simulink model "sensorFusionOffline"  (Simulink 7.8)
settings: Solver=FixedStepDiscrete  StartTime=0.0  StopTime=endTime  FixedStep=0.005  MaxStep=0.005  RelTol=1e-3
undefined symbols (not defined in the file or in its folder): EGOSF_CompassHeadingCov, EGOSF_DetectionNorthMax, EGOSF_DetectionNorthMin, EGOSF_HeadingVelocityLimit, EGOSF_LatAccCov, EGOSF_LonAccCov, EGOSF_LonSpeedCov, EGOSF_OutlierDetection, EGOSF_PhiCov, EGOSF_PhiScale, EGOSF_Pproc, EGOSF_SteeringRatio, EGOSF_UTMZone, EGOSF_YawRateCov
libraries: powerlib_meascontrol x1
settings Model: Creator=hultr  LastModifiedBy=mdv91
settings DataIOCC: SignalLoggingSaveFormat=Dataset
settings OptimizationCC: ExpressionDepthLimit=128
settings DebuggingCC: UnderspecifiedInitializationDetection=Simplified  MergeDetectMultiDrivingBlocksExec=error  InheritedTsInSrcMsg=none  BusObjectLabelMismatch=none  StateNameClashWarn=none
settings CodeAppCC: CustomSymbolStrType=$N$R$M_T
settings GRTTargetCC: TargetFunctionLibrary=C89/C90 (ANSI)

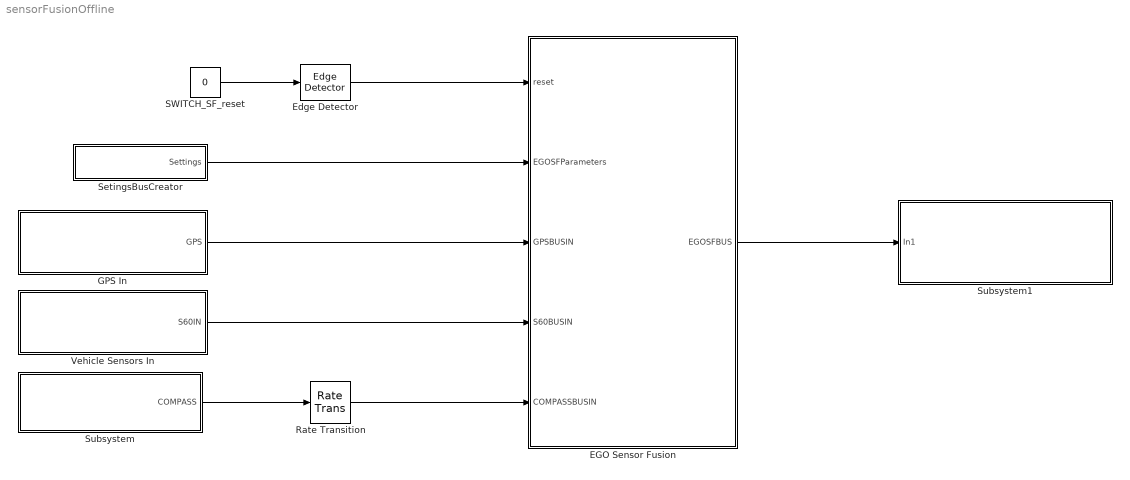
== system sensorFusionOffline ==
  EGO Sensor Fusion : MATLAB Function  TreatAsAtomicUnit=on  SystemSampleTime=0.025
      settings: PermitHierarchicalResolution=ParametersOnly
  Edge Detector : powerlib_meascontrol/Logic/Edge Detector  model=Rising  ic=0  Ts=-1
  GPS In : Subsystem
  Rate Transition : RateTransition
  SWITCH_SF_reset : Constant  Value=0  SampleTime=-1
  SetingsBusCreator : Subsystem
  Subsystem : Subsystem  TreatAsAtomicUnit=on  SystemSampleTime=0.1
  Subsystem1 : Subsystem
  Vehicle Sensors In : Subsystem
  wires:
  Subsystem/1("COMPASS ") -> Rate Transition/1
  GPS In/1(GPS) -> EGO Sensor Fusion/3(GPSBUSIN)
  Vehicle Sensors In/1(S60IN) -> EGO Sensor Fusion/4(S60BUSIN)
  SWITCH_SF_reset/1 -> Edge Detector/1
  SetingsBusCreator/1(Settings) -> EGO Sensor Fusion/2(EGOSFParameters)
  Rate Transition/1 -> EGO Sensor Fusion/5(COMPASSBUSIN)
  EGO Sensor Fusion/1(EGOSFBUS) -> Subsystem1/1(In1)
  Edge Detector/1 -> EGO Sensor Fusion/1(reset)

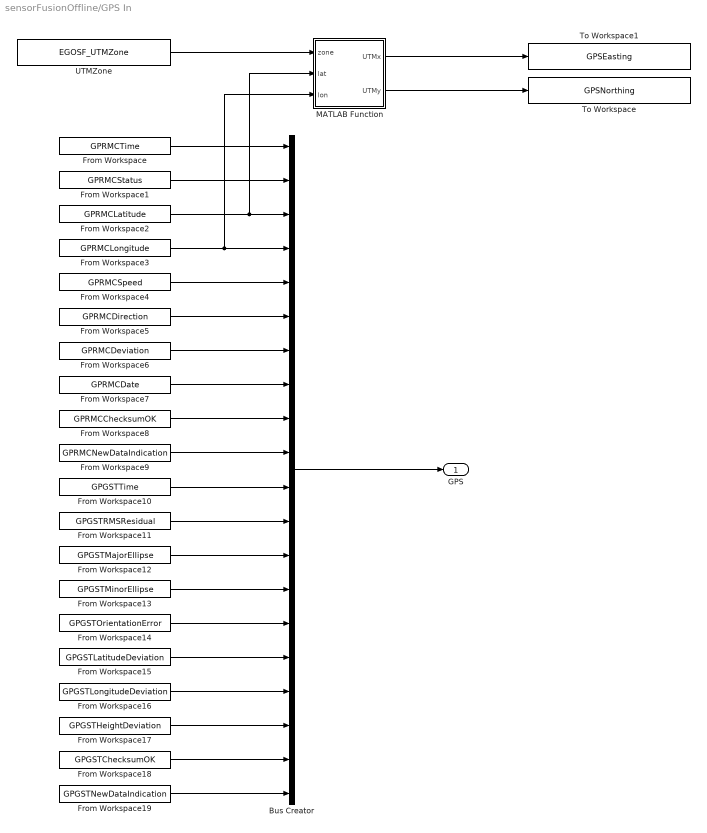
== system sensorFusionOffline/GPS In ==
  Bus Creator : BusCreator  Inputs=20  OutDataTypeStr=Bus: GPSBUS
  From Workspace : FromWorkspace  VariableName=GPRMCTime
  From Workspace1 : FromWorkspace  VariableName=GPRMCStatus
  From Workspace10 : FromWorkspace  VariableName=GPGSTTime
  From Workspace11 : FromWorkspace  VariableName=GPGSTRMSResidual
  From Workspace12 : FromWorkspace  VariableName=GPGSTMajorEllipse
  From Workspace13 : FromWorkspace  VariableName=GPGSTMinorEllipse
  From Workspace14 : FromWorkspace  VariableName=GPGSTOrientationError
  From Workspace15 : FromWorkspace  VariableName=GPGSTLatitudeDeviation
  From Workspace16 : FromWorkspace  VariableName=GPGSTLongitudeDeviation
  From Workspace17 : FromWorkspace  VariableName=GPGSTHeightDeviation
  From Workspace18 : FromWorkspace  VariableName=GPGSTChecksumOK
  From Workspace19 : FromWorkspace  VariableName=GPGSTNewDataIndication
  From Workspace2 : FromWorkspace  VariableName=GPRMCLatitude
  From Workspace3 : FromWorkspace  VariableName=GPRMCLongitude
  From Workspace4 : FromWorkspace  VariableName=GPRMCSpeed
  From Workspace5 : FromWorkspace  VariableName=GPRMCDirection
  From Workspace6 : FromWorkspace  VariableName=GPRMCDeviation
  From Workspace7 : FromWorkspace  VariableName=GPRMCDate
  From Workspace8 : FromWorkspace  VariableName=GPRMCChecksumOK
  From Workspace9 : FromWorkspace  VariableName=GPRMCNewDataIndication
  MATLAB Function : MATLAB Function  TreatAsAtomicUnit=on
      settings: PermitHierarchicalResolution=ParametersOnly
  To Workspace : ToWorkspace  VariableName=GPSNorthing  SaveFormat=Structure With Time  SampleTime=-1
  To Workspace1 : ToWorkspace  VariableName=GPSEasting  SaveFormat=Structure With Time  SampleTime=-1
  UTMZone : Constant  Value=EGOSF_UTMZone  SampleTime=-1
  GPS : Outport
  wires:
  From Workspace/1 -> Bus Creator/1
  Bus Creator/1 -> GPS/1
  From Workspace1/1 -> Bus Creator/2
  From Workspace2/1 -> MATLAB Function/2(lat), Bus Creator/3
  From Workspace3/1 -> MATLAB Function/3(lon), Bus Creator/4
  From Workspace4/1 -> Bus Creator/5
  From Workspace5/1 -> Bus Creator/6
  From Workspace6/1 -> Bus Creator/7
  From Workspace7/1 -> Bus Creator/8
  From Workspace8/1 -> Bus Creator/9
  From Workspace9/1 -> Bus Creator/10
  From Workspace10/1 -> Bus Creator/11
  From Workspace11/1 -> Bus Creator/12
  From Workspace12/1 -> Bus Creator/13
  From Workspace13/1 -> Bus Creator/14
  From Workspace14/1 -> Bus Creator/15
  From Workspace15/1 -> Bus Creator/16
  From Workspace16/1 -> Bus Creator/17
  From Workspace17/1 -> Bus Creator/18
  From Workspace18/1 -> Bus Creator/19
  From Workspace19/1 -> Bus Creator/20
  MATLAB Function/2(UTMy) -> To Workspace/1
  MATLAB Function/1(UTMx) -> To Workspace1/1
  UTMZone/1 -> MATLAB Function/1(zone)

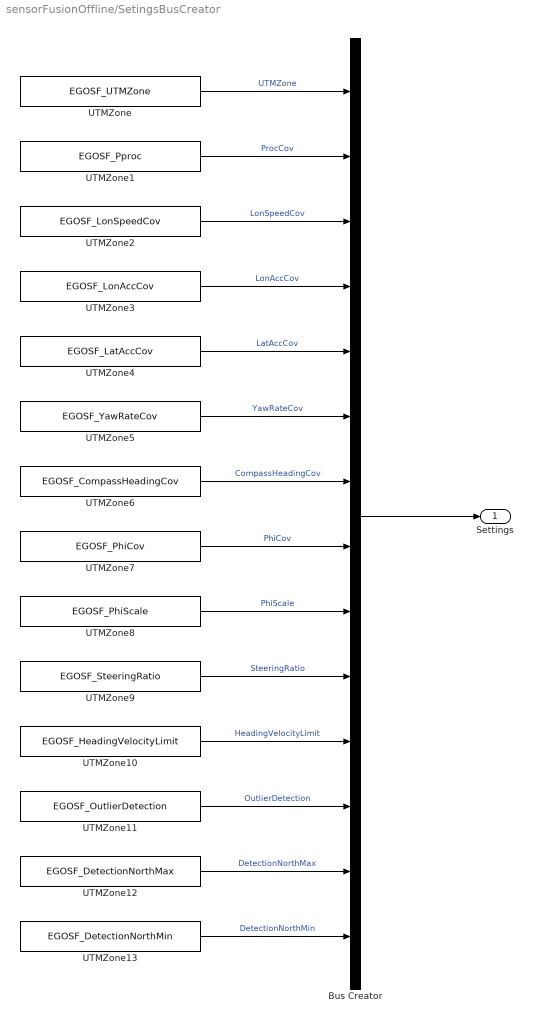
== system sensorFusionOffline/SetingsBusCreator ==
  Bus Creator : BusCreator  Inputs=14  OutDataTypeStr=Bus: EGOSFSETTINGS
  UTMZone : Constant  Value=EGOSF_UTMZone  SampleTime=-1
  UTMZone1 : Constant  Value=EGOSF_Pproc  SampleTime=-1
  UTMZone10 : Constant  Value=EGOSF_HeadingVelocityLimit  SampleTime=-1
  UTMZone11 : Constant  Value=EGOSF_OutlierDetection  SampleTime=-1
  UTMZone12 : Constant  Value=EGOSF_DetectionNorthMax  SampleTime=-1
  UTMZone13 : Constant  Value=EGOSF_DetectionNorthMin  SampleTime=-1
  UTMZone2 : Constant  Value=EGOSF_LonSpeedCov  SampleTime=-1
  UTMZone3 : Constant  Value=EGOSF_LonAccCov  SampleTime=-1
  UTMZone4 : Constant  Value=EGOSF_LatAccCov  SampleTime=-1
  UTMZone5 : Constant  Value=EGOSF_YawRateCov  SampleTime=-1
  UTMZone6 : Constant  Value=EGOSF_CompassHeadingCov  SampleTime=-1
  UTMZone7 : Constant  Value=EGOSF_PhiCov  SampleTime=-1
  UTMZone8 : Constant  Value=EGOSF_PhiScale  SampleTime=-1
  UTMZone9 : Constant  Value=EGOSF_SteeringRatio  SampleTime=-1
  Settings : Outport
  wires:
  Bus Creator/1 -> Settings/1
  UTMZone/1 -> Bus Creator/1  "UTMZone"
  UTMZone1/1 -> Bus Creator/2  "ProcCov"
  UTMZone2/1 -> Bus Creator/3  "LonSpeedCov"
  UTMZone3/1 -> Bus Creator/4  "LonAccCov"
  UTMZone5/1 -> Bus Creator/6  "YawRateCov"
  UTMZone6/1 -> Bus Creator/7  "CompassHeadingCov"
  UTMZone4/1 -> Bus Creator/5  "LatAccCov"
  UTMZone7/1 -> Bus Creator/8  "PhiCov"
  UTMZone8/1 -> Bus Creator/9  "PhiScale"
  UTMZone9/1 -> Bus Creator/10  "SteeringRatio"
  UTMZone10/1 -> Bus Creator/11  "HeadingVelocityLimit"
  UTMZone11/1 -> Bus Creator/12  "OutlierDetection"
  UTMZone12/1 -> Bus Creator/13  "DetectionNorthMax"
  UTMZone13/1 -> Bus Creator/14  "DetectionNorthMin"

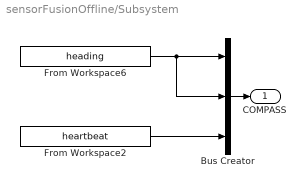
== system sensorFusionOffline/Subsystem ==
  Bus Creator : BusCreator  Inputs=3  OutDataTypeStr=Bus: COMPASSBUS
  From Workspace2 : FromWorkspace  VariableName=heartbeat
  From Workspace6 : FromWorkspace  VariableName=heading
  "COMPASS " : Outport
  wires:
  From Workspace2/1 -> Bus Creator/3
  From Workspace6/1 -> Bus Creator/2, Bus Creator/1
  Bus Creator/1 -> "COMPASS "/1

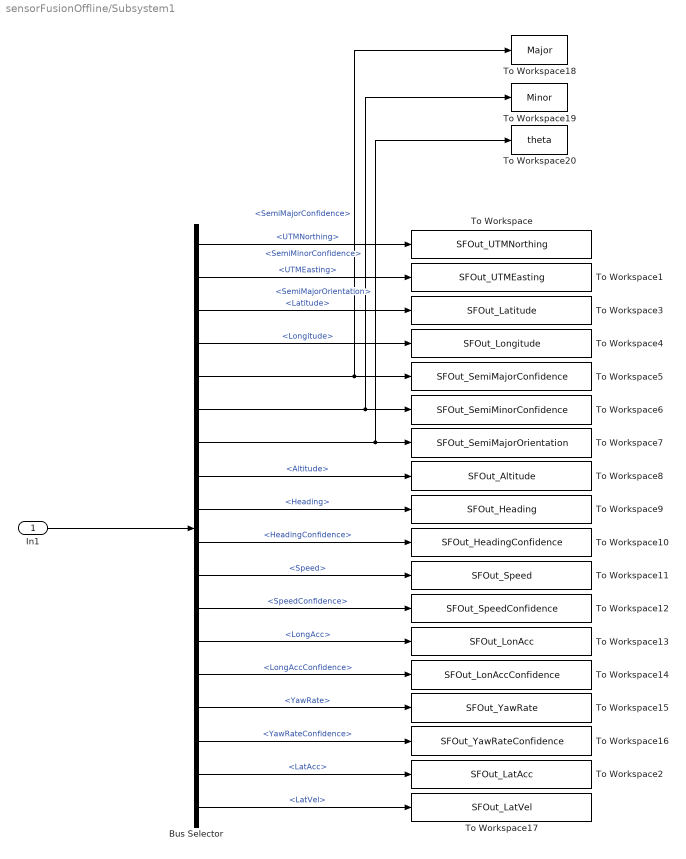
== system sensorFusionOffline/Subsystem1 ==
  In1 : Inport
  Bus Selector : BusSelector  OutputSignals=UTMNorthing,UTMEasting,Latitude,Longitude,SemiMajorConfidence,SemiMinorConfidence,SemiMajorOrientation,Altitude,Heading,HeadingConfidence,Speed,SpeedConfidence,LongAcc,LongAccConfidence,YawRate,YawRateConfidence,LatAcc,LatVel
  To Workspace : ToWorkspace  VariableName=SFOut_UTMNorthing  SaveFormat=Structure With Time  SampleTime=-1
  To Workspace1 : ToWorkspace  VariableName=SFOut_UTMEasting  SaveFormat=Structure With Time  SampleTime=-1
  To Workspace10 : ToWorkspace  VariableName=SFOut_HeadingConfidence  SaveFormat=Structure With Time  SampleTime=-1
  To Workspace11 : ToWorkspace  VariableName=SFOut_Speed  SaveFormat=Structure With Time  SampleTime=-1
  To Workspace12 : ToWorkspace  VariableName=SFOut_SpeedConfidence  SaveFormat=Structure With Time  SampleTime=-1
  To Workspace13 : ToWorkspace  VariableName=SFOut_LonAcc  SaveFormat=Structure With Time  SampleTime=-1
  To Workspace14 : ToWorkspace  VariableName=SFOut_LonAccConfidence  SaveFormat=Structure With Time  SampleTime=-1
  To Workspace15 : ToWorkspace  VariableName=SFOut_YawRate  SaveFormat=Structure With Time  SampleTime=-1
  To Workspace16 : ToWorkspace  VariableName=SFOut_YawRateConfidence  SaveFormat=Structure With Time  SampleTime=-1
  To Workspace17 : ToWorkspace  VariableName=SFOut_LatVel  SaveFormat=Structure With Time  SampleTime=-1
  To Workspace18 : ToWorkspace  VariableName=Major  SaveFormat=Structure With Time  SampleTime=-1
  To Workspace19 : ToWorkspace  VariableName=Minor  SaveFormat=Structure With Time  SampleTime=-1
  To Workspace2 : ToWorkspace  VariableName=SFOut_LatAcc  SaveFormat=Structure With Time  SampleTime=-1
  To Workspace20 : ToWorkspace  VariableName=theta  SaveFormat=Structure With Time  SampleTime=-1
  To Workspace3 : ToWorkspace  VariableName=SFOut_Latitude  SaveFormat=Structure With Time  SampleTime=-1
  To Workspace4 : ToWorkspace  VariableName=SFOut_Longitude  SaveFormat=Structure With Time  SampleTime=-1
  To Workspace5 : ToWorkspace  VariableName=SFOut_SemiMajorConfidence  SaveFormat=Structure With Time  SampleTime=-1
  To Workspace6 : ToWorkspace  VariableName=SFOut_SemiMinorConfidence  SaveFormat=Structure With Time  SampleTime=-1
  To Workspace7 : ToWorkspace  VariableName=SFOut_SemiMajorOrientation  SaveFormat=Structure With Time  SampleTime=-1
  To Workspace8 : ToWorkspace  VariableName=SFOut_Altitude  SaveFormat=Structure With Time  SampleTime=-1
  To Workspace9 : ToWorkspace  VariableName=SFOut_Heading  SaveFormat=Structure With Time  SampleTime=-1
  wires:
  In1/1 -> Bus Selector/1
  Bus Selector/1 -> To Workspace/1  "<UTMNorthing>"
  Bus Selector/2 -> To Workspace1/1  "<UTMEasting>"
  Bus Selector/3 -> To Workspace3/1  "<Latitude>"
  Bus Selector/4 -> To Workspace4/1  "<Longitude>"
  Bus Selector/5 -> To Workspace18/1, To Workspace5/1  "<SemiMajorConfidence>"
  Bus Selector/6 -> To Workspace19/1, To Workspace6/1  "<SemiMinorConfidence>"
  Bus Selector/7 -> To Workspace20/1, To Workspace7/1  "<SemiMajorOrientation>"
  Bus Selector/8 -> To Workspace8/1  "<Altitude>"
  Bus Selector/9 -> To Workspace9/1  "<Heading>"
  Bus Selector/10 -> To Workspace10/1  "<HeadingConfidence>"
  Bus Selector/11 -> To Workspace11/1  "<Speed>"
  Bus Selector/12 -> To Workspace12/1  "<SpeedConfidence>"
  Bus Selector/13 -> To Workspace13/1  "<LongAcc>"
  Bus Selector/14 -> To Workspace14/1  "<LongAccConfidence>"
  Bus Selector/15 -> To Workspace15/1  "<YawRate>"
  Bus Selector/16 -> To Workspace16/1  "<YawRateConfidence>"
  Bus Selector/17 -> To Workspace2/1  "<LatAcc>"
  Bus Selector/18 -> To Workspace17/1  "<LatVel>"

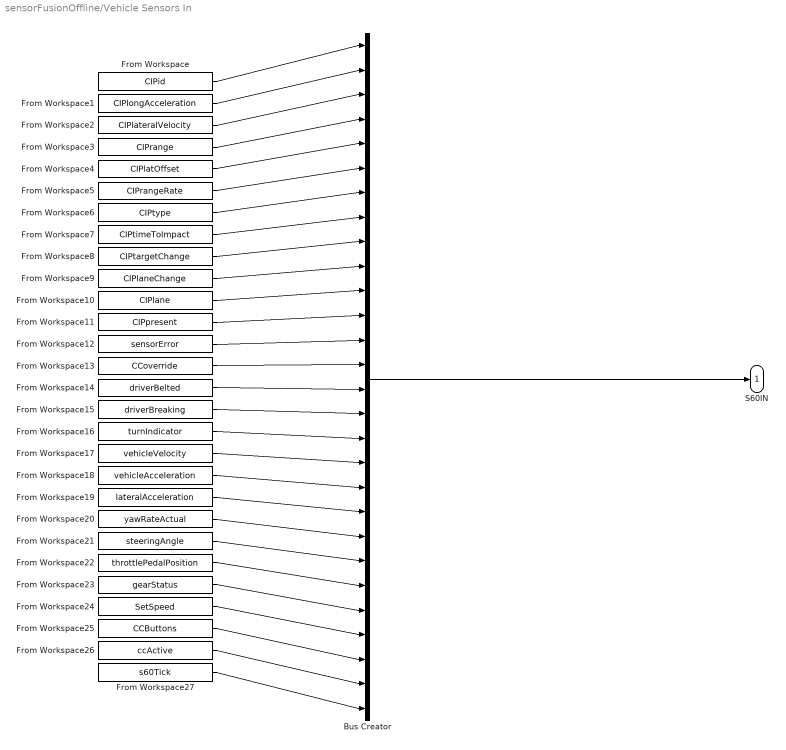
== system sensorFusionOffline/Vehicle Sensors In ==
  Bus Creator : BusCreator  Inputs=28  OutDataTypeStr=Bus: S60OUTBUS
  From Workspace : FromWorkspace  VariableName=CIPid
  From Workspace1 : FromWorkspace  VariableName=CIPlongAcceleration
  From Workspace10 : FromWorkspace  VariableName=CIPlane
  From Workspace11 : FromWorkspace  VariableName=CIPpresent
  From Workspace12 : FromWorkspace  VariableName=sensorError
  From Workspace13 : FromWorkspace  VariableName=CCoverride
  From Workspace14 : FromWorkspace  VariableName=driverBelted
  From Workspace15 : FromWorkspace  VariableName=driverBreaking
  From Workspace16 : FromWorkspace  VariableName=turnIndicator
  From Workspace17 : FromWorkspace  VariableName=vehicleVelocity
  From Workspace18 : FromWorkspace  VariableName=vehicleAcceleration
  From Workspace19 : FromWorkspace  VariableName=lateralAcceleration
  From Workspace2 : FromWorkspace  VariableName=CIPlateralVelocity
  From Workspace20 : FromWorkspace  VariableName=yawRateActual
  From Workspace21 : FromWorkspace  VariableName=steeringAngle
  From Workspace22 : FromWorkspace  VariableName=throttlePedalPosition
  From Workspace23 : FromWorkspace  VariableName=gearStatus
  From Workspace24 : FromWorkspace  VariableName=SetSpeed
  From Workspace25 : FromWorkspace  VariableName=CCButtons
  From Workspace26 : FromWorkspace  VariableName=ccActive
  From Workspace27 : FromWorkspace  VariableName=s60Tick
  From Workspace3 : FromWorkspace  VariableName=CIPrange
  From Workspace4 : FromWorkspace  VariableName=CIPlatOffset
  From Workspace5 : FromWorkspace  VariableName=CIPrangeRate
  From Workspace6 : FromWorkspace  VariableName=CIPtype
  From Workspace7 : FromWorkspace  VariableName=CIPtimeToImpact
  From Workspace8 : FromWorkspace  VariableName=CIPtargetChange
  From Workspace9 : FromWorkspace  VariableName=CIPlaneChange
  S60IN : Outport
  wires:
  Bus Creator/1 -> S60IN/1
  From Workspace/1 -> Bus Creator/1
  From Workspace1/1 -> Bus Creator/2
  From Workspace2/1 -> Bus Creator/3
  From Workspace3/1 -> Bus Creator/4
  From Workspace4/1 -> Bus Creator/5
  From Workspace5/1 -> Bus Creator/6
  From Workspace6/1 -> Bus Creator/7
  From Workspace7/1 -> Bus Creator/8
  From Workspace8/1 -> Bus Creator/9
  From Workspace9/1 -> Bus Creator/10
  From Workspace10/1 -> Bus Creator/11
  From Workspace11/1 -> Bus Creator/12
  From Workspace13/1 -> Bus Creator/14
  From Workspace12/1 -> Bus Creator/13
  From Workspace23/1 -> Bus Creator/24
  From Workspace17/1 -> Bus Creator/18
  From Workspace18/1 -> Bus Creator/19
  From Workspace20/1 -> Bus Creator/21
  From Workspace21/1 -> Bus Creator/22
  From Workspace16/1 -> Bus Creator/17
  From Workspace15/1 -> Bus Creator/16
  From Workspace25/1 -> Bus Creator/26
  From Workspace19/1 -> Bus Creator/20
  From Workspace24/1 -> Bus Creator/25
  From Workspace14/1 -> Bus Creator/15
  From Workspace22/1 -> Bus Creator/23
  From Workspace26/1 -> Bus Creator/27
  From Workspace27/1 -> Bus Creator/28

== matlab function EGO Sensor Fusion ==
  data: reset input double; EGOSFParameters input Bus: EGOSFSETTINGS; GPSBUSIN input Bus: GPSBUS; EGOSFBUS output Bus: EGOSFBUS; S60BUSIN input Bus: S60OUTBUS; COMPASSBUSIN input Bus: COMPASSBUS
function EGOSFBUS = fcn(reset,EGOSFParameters,GPSBUSIN,S60BUSIN,COMPASSBUSIN)
%#codegen
% =========================================================================
% GCDC Sensor fusion offline template. Modify as needed
% Robert Hult, 10/3-16
%
% SOME RECOMMENDATIONS:
%  - in the update steps, build the measurment equations "on the fly"
%    depending on which sensors has new data
%  - Include a validity-check on the GPS data, outliers are relatively
%    common, especially when using the correction
%  - Take care with angles! be aware that things might get weird du to mod
%    2Pi. This MUST be handled in some waym otherwsie we will get weird
%    behaviour.
%  - NOTE: All measurments are NOT given in SI units
%
% =========================================================================
% Dummy example implementation using unicycle kinematics
% State X = [x,y,vlon,alon,vlat,alat,yaw,yawrate,phi]
nStates = 9;
persistent X 
if isempty(X)
    X = zeros(nStates,1);
%     X(3) = S60BUSIN.vehicleVelocity;
%     X(4) = S60BUSIN.vehicleAcceleration;
%     X(5) = 0;
%     X(6) = S60BUSIN.lateralAcceleration;
%     X(7) = COMPASSBUSIN.heading;
%     X(8) = S60BUSIN.yawRateActual;
%     X(9) = 0;
end

persistent P
if isempty(P)
    P = zeros(nStates);
end

%%%%%%%%%%%%%%%%%%%%%%%%%%%%%%%%%%%%%%%%%%%%%%%%%%%%%%%%%%%%%%%%%%%%%%%%%%%
%%%%%%%%%%%%%%%%%%%% DATA CHECKING %%%%%%%%%%%%%%%%%%%%%%%%%%%%%%%%%%%%%%%%
%%%%%%%%%%%%%%%%%%%%%%%%%%%%%%%%%%%%%%%%%%%%%%%%%%%%%%%%%%%%%%%%%%%%%%%%%%%
% CHECK GPS DATA
persistent timeAtPreviousGPSreading
if isempty(timeAtPreviousGPSreading)
    timeAtPreviousGPSreading = 0;
end

if GPSBUSIN.GPRMCTime == timeAtPreviousGPSreading || GPSBUSIN.GPRMCStatus ~= 1
   UTMx             = NaN;
   UTMy             = NaN;
   GpsCov           = NaN(2);
   newGPSData       = 0;
else
% FUNCTIONS FOUND IN AUXILARY FOLDER
% Decimal degrees to DEG,Min,sec.decsec
[Latdec,Londec]= dm2deg(GPSBUSIN.GPRMCLatitude,GPSBUSIN.GPRMCLongitude);
% Decimal degrees to UTM approximation
[UTMx, UTMy] = wgs2utm(Latdec,Londec,EGOSFParameters.UTMZone);
% Convert Covariance
GpsCov=gpscov(GPSBUSIN.GPGSTMajorEllipse,GPSBUSIN.GPGSTMinorEllipse,GPSBUSIN.GPGSTOrientationError);
newGPSData = 1;
end


% =========================================================================
% =========================================================================
% CHECK S60 DATA
persistent tickAtPreviousS60Reading
if isempty(tickAtPreviousS60Reading)
    tickAtPreviousS60Reading = 0;
end

if tickAtPreviousS60Reading ~= S60BUSIN.s60Tick
    tickAtPreviousS60Reading = S60BUSIN.s60Tick;
    newS60Data = 1;
else
    newS60Data = 0;
end

% =========================================================================
% =========================================================================
% CHECK COMPASS DATA
persistent tickAtPreviousCompassReading
if isempty(tickAtPreviousCompassReading)
    tickAtPreviousCompassReading = 0;
end

if tickAtPreviousCompassReading ~= COMPASSBUSIN.heartbeat
    tickAtPreviousCompassReading = COMPASSBUSIN.heartbeat;
    newCompassData = 1;
else
    newCompassData = 0;
end

%%%%%%%%%%%%%%%%%%%%%%%%%%%%%%%%%%%%%%%%%%%%%%%%%%%%%%%%%%%%%%%%%%%%%%%%%%%
%%%%%%%%%%%%%%%% FILTER MANAGEMENT LOGIC  %%%%%%%%%%%%%%%%%%%%%%%%%%%%%%%%%
%%%%%%%%%%%%%%%%%%%%%%%%%%%%%%%%%%%%%%%%%%%%%%%%%%%%%%%%%%%%%%%%%%%%%%%%%%%
% 1) Enables resetting of state and covariances
% 2) Initializes the states as the sensor values on reset.
% 3) Initializes the position when new GPS data comes in, otherwise freezes
%    it on the last recieved position (completely arbitrary)
%
% -------------------------------------------------------------------------
persistent positionIsInitialized
if isempty(positionIsInitialized)
   positionIsInitialized = 0; 
end

if reset == 1
   % Reset State, reset covariance
   X = X*0;
   X(3) = S60BUSIN.vehicleVelocity;
   X(4) = S60BUSIN.vehicleAcceleration;
   X(5) = 0;
   X(6) = S60BUSIN.lateralAcceleration;
   X(7) = GPSBUSIN.GPRMCDirection;
   X(8) = S60BUSIN.yawRateActual;
   X(9) = 0;
    
    
elseif ~positionIsInitialized
    if newGPSData
        if S60BUSIN.vehicleVelocity > 10
            %(5) 
        end
        positionIsInitialized = 1;       
    end
    X(1) = UTMx;
    X(2) = UTMy;
end

%%%%%%%%%%%%%%%%%%%%%%%%%%%%%%%%%%%%%%%%%%%%%%%%%%%%%%%%%%%%%%%%%%%%%%%%%%%
%%%%%%%%%%%%%%%%%%%%% PREDICTION-CORRECTION %%%%%%%%%%%%%%%%%%%%%%%%%%%%%%%
%%%%%%%%%%%%%%%%%%%%%%%%%%%%%%%%%%%%%%%%%%%%%%%%%%%%%%%%%%%%%%%%%%%%%%%%%%%

% PREDICTION

if abs(X(3))<0.01
    X(3)=0.01;
end

X  = dynamicsFun(X);
dF = jacobianFun(X); 
P  =  dF*P*dF' + EGOSFParameters.ProcCov;

% CORRECTION (Assumption is that vehicle allways give new data)

yMeasured  = [UTMx; UTMy; S60BUSIN.vehicleVelocity; S60BUSIN.vehicleAcceleration; S60BUSIN.lateralAcceleration; (2*pi -GPSBUSIN.GPRMCDirection*pi/180); S60BUSIN.yawRateActual*pi/180; +(S60BUSIN.steeringAngle*pi/180)/EGOSFParameters.SteeringRatio  ]; % -(COMPASSBUSIN.heading)+2*pi  GPSBUSIN.GPRMCDirection*pi/180 -(2*pi -GPSBUSIN.GPRMCDirection*pi/180)
tmp = eye(9);
I = [(1:4),(6:9)];
H = tmp(I,:);
H(8,9) = EGOSFParameters.PhiScale;

yEstimate  = H*X; 

Rconst = diag([EGOSFParameters.LonSpeedCov,...
               EGOSFParameters.LonAccCov,...
               EGOSFParameters.LatAccCov,...
               EGOSFParameters.CompassHeadingCov,...
               EGOSFParameters.YawRateCov,...            %EGOSFParameters.CompassHeadingCov 0.1*GPSBUSIN.GPGSTOrientationError*pi/180
               EGOSFParameters.PhiCov]);

R = blkdiag(GpsCov,Rconst);


X_e = [ yEstimate(1)-yMeasured(1); yEstimate(2)-yMeasured(2)];                              %Error of position

if newGPSData
    
    if S60BUSIN.vehicleVelocity >= EGOSFParameters.HeadingVelocityLimit 
        I = 1:8;
    else
        I = [1,2,3,4,5,7,8];
    end
    
    if sqrt(X_e'*X_e)>EGOSFParameters.OutlierDetection  %X_e'/(P(1:2,1:2))*X_e>2
        I=I(3:end);
    end
    
else
    I = [3,4,5,6,8];
end

up = 0;
if newGPSData && X(7)>EGOSFParameters.DetectionNorthMax && yMeasured(6)<EGOSFParameters.DetectionNorthMin
    yMeasured(6) = 2*pi + yMeasured(6);
    up=1;
elseif newGPSData && X(7)<EGOSFParameters.DetectionNorthMin && yMeasured(6)>EGOSFParameters.DetectionNorthMax
    yMeasured(6) = -2*pi + yMeasured(6);
    up=1;
end

innovation = yMeasured(I)-yEstimate(I); 

S = H(I,:)*P*(H(I,:))' + R(I,I);

K = P*(H(I,:)'/S);
X = X + K*innovation;
P = (eye(nStates) - K*H(I,:))*P;

if up==1
    X(7) = mod(X(7),2*pi);
end

%%%%%%%%%%%%%%%%%%%%%%%%%%%%%%%%%%%%%%%%%%%%%%%%%%%%%%%%%%%%%%%%%%%%%%%%%%%
%%%%%%%%%%%%%%%%%%%%% OUTPUT FORMATTING %%%%%%%%%%%%%%%%%%%%%%%%%%%%%%%%%%%
%%%%%%%%%%%%%%%%%%%%%%%%%%%%%%%%%%%%%%%%%%%%%%%%%%%%%%%%%%%%%%%%%%%%%%%%%%%
% NOTE THAT SIGNALS MUCH BE DEFINED IN THE ORDER IT APPEARS IN THE BUS

[Lat,Lon]=utm2wgs(X(1),X(2),EGOSFParameters.UTMZone);
[SemiMajor,SemiMinor,Theta]= errorEllips(P(1:2,1:2));

EGOSFBUS.UTMNorthing            = X(2);
EGOSFBUS.UTMEasting             = X(1);
EGOSFBUS.Latitude               = Lat; % Dont forget
EGOSFBUS.Longitude              = Lon; % Dont forget
EGOSFBUS.SemiMajorConfidence 	= SemiMajor; % Dont forget
EGOSFBUS.SemiMinorConfidence    = SemiMinor; % Dont forget
EGOSFBUS.SemiMajorOrientation   = Theta; % Dont forget
EGOSFBUS.Altitude               = 0; % Dont forget
EGOSFBUS.Heading                = X(7);
EGOSFBUS.HeadingConfidence      = P(7,7);
EGOSFBUS.Speed                  = X(3);
EGOSFBUS.SpeedConfidence        = P(3,3);
EGOSFBUS.LongAcc                = X(4);
EGOSFBUS.LongAccConfidence      = P(4,4);
EGOSFBUS.YawRate                = X(8);
EGOSFBUS.YawRateConfidence      = P(8,8);
EGOSFBUS.LatAcc                 = X(6); % Dont forget
EGOSFBUS.LatVel                 = X(5); % Dont forget
end

== matlab function GPS In/MATLAB Function ==
  data: zone input double; UTMx output double; lat input double; UTMy output double; lon input double
function [UTMx,UTMy] = fcn(zone,lat,lon)
%#codegen


[Latdec,Londec]= dm2deg(lat,lon);
% Decimal degrees to UTM approximation
[UTMx, UTMy] = wgs2utm(Latdec,Londec,zone);
